simulink model "trajgen2_ste2_realtraj"  (R2016a)
settings: Solver=FixedStepDiscrete  StartTime=0.0  StopTime=10  RelTol=1e-3
undefined symbols (not defined in the file or in its folder): min_dist, robot_trajectory_data, robot_trajectory_s, start_time, THumanSingleTask
settings Model: Creator=ihout_000  LastModifiedBy=utente
settings DataIOCC: SaveFormat=Array
settings OptimizationCC: ExpressionDepthLimit=2147483647  SimCompilerOptimization=on
settings DebuggingCC: UnderspecifiedInitializationDetection=Classic  MergeDetectMultiDrivingBlocksExec=none  SolverPrmCheckMsg=warning  InheritedTsInSrcMsg=none  StateNameClashWarn=warning
settings HardwareCC: ProdBitPerPointer=32  ProdLargestAtomicFloat=None  ProdIntDivRoundTo=Undefined  ProdEndianess=Unspecified  ProdWordSize=32  ProdHWDeviceType=32-bit Generic
settings ModelReferenceCC: PropagateSignalLabelsOutOfModel=off
settings SFSimCC: SimUserIncludeDirs=ReflexxesTypeII\include\
settings SFSimCC: SimUserSources=|
  | ReflexxesTypeII\src\TypeIIRML\ReflexxesAPI.cpp
  | ReflexxesTypeII\src\TypeIIRML\TypeIIRMLCalculatePositionalExtrems.cpp
  | ReflexxesTypeII\src\TypeIIRML\TypeIIRMLDecisions.cpp
  | ReflexxesTypeII\src\TypeIIRML\TypeIIRMLDecisionTree1A.cpp
  | ReflexxesTypeII\src\TypeIIRML\TypeIIRMLDecisionTree1B.cpp
  | ReflexxesTypeII\src\TypeIIRML\TypeIIRMLDecisionTree1C.cpp
  | ReflexxesTypeII\src\TypeIIRML\TypeIIRMLDecisionTree2.cpp
  | ReflexxesTypeII\src\TypeIIRML\TypeIIRMLFallBackStrategy.cpp
  | ReflexxesTypeII\src\TypeIIRML\TypeIIRMLIsPhaseSynchronizationPossible.cpp
  | ReflexxesTypeII\src\TypeIIRML\TypeIIRMLPolynomial.cpp
  | ReflexxesTypeII\src\TypeIIRML\TypeIIRMLPosition.cpp
  | ReflexxesTypeII\src\TypeIIRML\TypeIIRMLQuicksort.cpp
  | ReflexxesTypeII\src\TypeIIRML\TypeIIRMLSetupModifiedSelectionVector.cpp
  | ReflexxesTypeII\src\TypeIIRML\TypeIIRMLStep1.cpp
  | ReflexxesTypeII\src\TypeIIRML\TypeIIRMLStep1IntermediateProfiles.cpp
  | ReflexxesTypeII\src\TypeIIRML\TypeIIRMLStep1Profiles.cpp
  | ReflexxesTypeII\src\TypeIIRML\TypeIIRMLStep2.cpp
  | ReflexxesTypeII\src\TypeIIRML\TypeIIRMLStep2IntermediateProfiles.cpp
  | ReflexxesTypeII\src\TypeIIRML\TypeIIRMLStep2PhaseSynchronization.cpp
  | ReflexxesTypeII\src\TypeIIRML\TypeIIRMLStep2Profiles.cpp
  | ReflexxesTypeII\src\TypeIIRML\TypeIIRMLStep2WithoutSynchronization.cpp
  | ReflexxesTypeII\src\TypeIIRML\TypeIIRMLStep3.cpp
  | ReflexxesTypeII\src\TypeIIRML\TypeIIRMLVelocity.cpp
  | ReflexxesTypeII\src\TypeIIRML\TypeIIRMLVelocityCalculatePositionalExtrems.cpp
  | ReflexxesTypeII\src\TypeIIRML\TypeIIRMLVelocityFallBackStrategy.cpp
  | ReflexxesTypeII\src\TypeIIRML\TypeIIRMLVelocityIsPhaseSynchronizationPossible.cpp
  | ReflexxesTypeII\src\TypeIIRML\TypeIIRMLVelocityMethods.cpp
  | ReflexxesTypeII\src\TypeIIRML\TypeIIRMLVelocitySetupPhaseSyncSelectionVector.cpp
settings RTWCC: GenerateMakefile=off  CustomInclude=ReflexxesTypeII\include\  TargetLang=C++  RTWCompilerOptimization=on
settings RTWCC: CustomSource=|
  | ReflexxesTypeII\src\TypeIIRML\ReflexxesAPI.cpp
  | ReflexxesTypeII\src\TypeIIRML\TypeIIRMLCalculatePositionalExtrems.cpp
  | ReflexxesTypeII\src\TypeIIRML\TypeIIRMLDecisions.cpp
  | ReflexxesTypeII\src\TypeIIRML\TypeIIRMLDecisionTree1A.cpp
  | ReflexxesTypeII\src\TypeIIRML\TypeIIRMLDecisionTree1B.cpp
  | ReflexxesTypeII\src\TypeIIRML\TypeIIRMLDecisionTree1C.cpp
  | ReflexxesTypeII\src\TypeIIRML\TypeIIRMLDecisionTree2.cpp
  | ReflexxesTypeII\src\TypeIIRML\TypeIIRMLFallBackStrategy.cpp
  | ReflexxesTypeII\src\TypeIIRML\TypeIIRMLIsPhaseSynchronizationPossible.cpp
  | ReflexxesTypeII\src\TypeIIRML\TypeIIRMLPolynomial.cpp
  | ReflexxesTypeII\src\TypeIIRML\TypeIIRMLPosition.cpp
  | ReflexxesTypeII\src\TypeIIRML\TypeIIRMLQuicksort.cpp
  | ReflexxesTypeII\src\TypeIIRML\TypeIIRMLSetupModifiedSelectionVector.cpp
  | ReflexxesTypeII\src\TypeIIRML\TypeIIRMLStep1.cpp
  | ReflexxesTypeII\src\TypeIIRML\TypeIIRMLStep1IntermediateProfiles.cpp
  | ReflexxesTypeII\src\TypeIIRML\TypeIIRMLStep1Profiles.cpp
  | ReflexxesTypeII\src\TypeIIRML\TypeIIRMLStep2.cpp
  | ReflexxesTypeII\src\TypeIIRML\TypeIIRMLStep2IntermediateProfiles.cpp
  | ReflexxesTypeII\src\TypeIIRML\TypeIIRMLStep2PhaseSynchronization.cpp
  | ReflexxesTypeII\src\TypeIIRML\TypeIIRMLStep2Profiles.cpp
  | ReflexxesTypeII\src\TypeIIRML\TypeIIRMLStep2WithoutSynchronization.cpp
  | ReflexxesTypeII\src\TypeIIRML\TypeIIRMLStep3.cpp
  | ReflexxesTypeII\src\TypeIIRML\TypeIIRMLVelocity.cpp
  | ReflexxesTypeII\src\TypeIIRML\TypeIIRMLVelocityCalculatePositionalExtrems.cpp
  | ReflexxesTypeII\src\TypeIIRML\TypeIIRMLVelocityFallBackStrategy.cpp
  | ReflexxesTypeII\src\TypeIIRML\TypeIIRMLVelocityIsPhaseSynchronizationPossible.cpp
  | ReflexxesTypeII\src\TypeIIRML\TypeIIRMLVelocityMethods.cpp
  | ReflexxesTypeII\src\TypeIIRML\TypeIIRMLVelocitySetupPhaseSyncSelectionVector.cpp
settings GRTTargetCC: TargetLangStandard=C++03 (ISO)
settings ConfigComp: CovModelRefEnable=Off

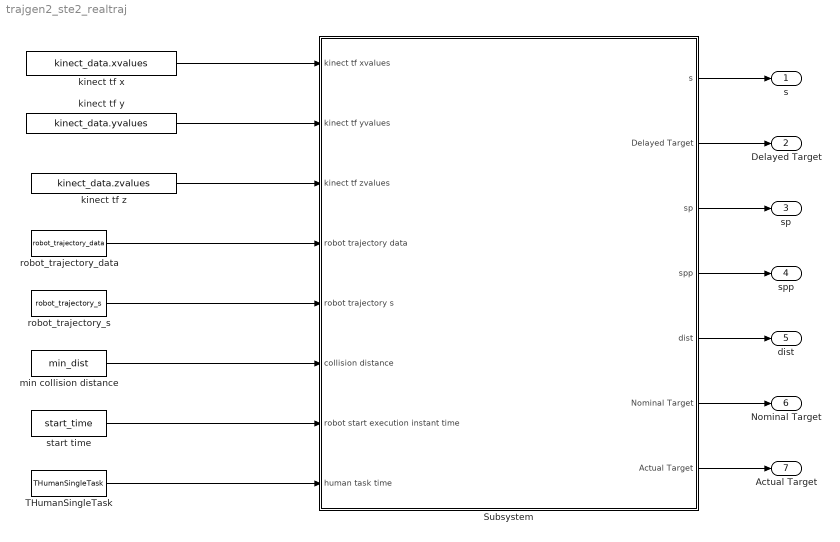
== system trajgen2_ste2_realtraj ==
  Subsystem : Subsystem
  THumanSingleTask : Constant  Value=THumanSingleTask
  kinect tf x : FromWorkspace  VariableName=kinect_data.xvalues  OutDataTypeStr=double
  kinect tf y : FromWorkspace  VariableName=kinect_data.yvalues  SampleTime=0
  kinect tf z : FromWorkspace  VariableName=kinect_data.zvalues  SampleTime=0
  min collision distance : Constant  Value=min_dist
  robot_trajectory_data : Constant  Value=robot_trajectory_data
  robot_trajectory_s : Constant  Value=robot_trajectory_s
  start time : Constant  Value=start_time
  s : Outport
  "Delayed Target " : Outport  Port=2
  sp : Outport  Port=3
  spp : Outport  Port=4
  dist : Outport  Port=5
  Nominal Target : Outport  Port=6
  Actual Target : Outport  Port=7
  wires:
  Subsystem/1(s) -> s/1
  kinect tf x/1 -> Subsystem/1("kinect tf xvalues ")
  kinect tf z/1 -> Subsystem/3(kinect tf zvalues)
  kinect tf y/1 -> Subsystem/2(kinect tf yvalues)
  Subsystem/2("Delayed Target ") -> "Delayed Target "/1
  robot_trajectory_data/1 -> Subsystem/4(robot trajectory data)
  robot_trajectory_s/1 -> Subsystem/5(robot trajectory s)
  Subsystem/5(dist) -> dist/1
  Subsystem/3(sp) -> sp/1
  Subsystem/4(spp) -> spp/1
  min collision distance/1 -> Subsystem/6(collision distance)
  Subsystem/6(Nominal Target) -> Nominal Target/1
  Subsystem/7(Actual Target) -> Actual Target/1
  start time/1 -> Subsystem/7(robot start execution instant time)
  THumanSingleTask/1 -> Subsystem/8("human task time ")

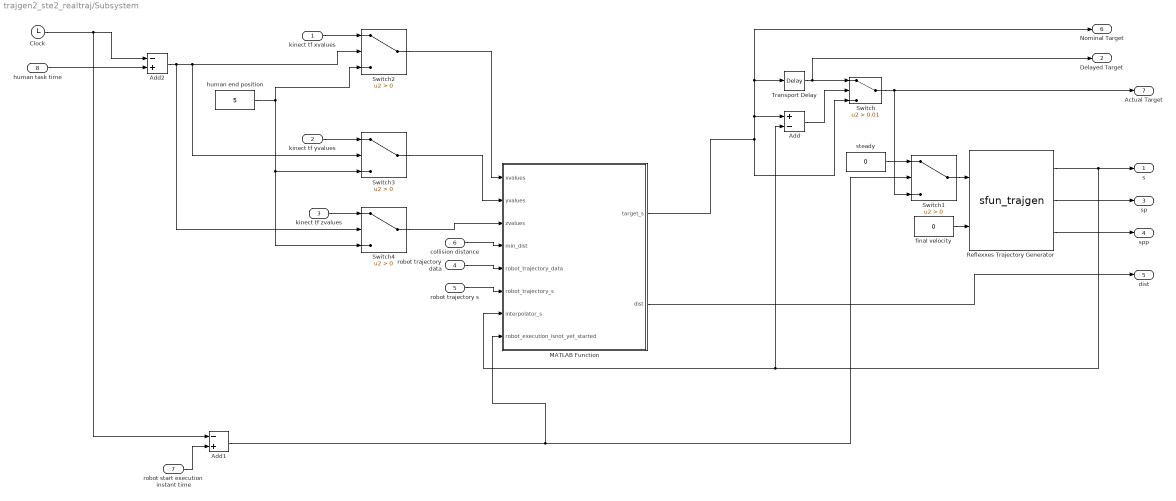
== system trajgen2_ste2_realtraj/Subsystem ==
  "kinect tf xvalues " : Inport
  kinect tf yvalues : Inport  Port=2
  kinect tf zvalues : Inport  Port=3
  robot trajectory data : Inport  Port=4
  robot trajectory s : Inport  Port=5
  collision distance : Inport  Port=6
  robot start execution instant time : Inport  Port=7
  "human task time " : Inport  Port=8
  Add : Sum  Inputs=+-
  Add1 : Sum  Inputs=-+
  Add2 : Sum  Inputs=-+
  Clock : Clock
  MATLAB Function : MATLAB Function  TreatAsAtomicUnit=on
  Reflexxes Trajectory Generator : S-Function  FunctionName=sfun_trajgen  Parameters=ts,ndofs,pinit,vmax,amax,jmax,sync  SFunctionDeploymentMode=off  EnableBusSupport=off  mask{ts=0.005, ndofs=1, pinit=0, vmax=0.250, amax=0.115, jmax=10000000000, sync=PHASE_SYNCHRONIZATION_IF_POSSIBLE}
      mask prompts: ts "Sample Time:"; ndofs "Number of DoF's:"; pinit "Initial Position Vector:"; vmax "Maximum Velocity Vector:"; amax "Maximum Acceleration Vector:"; jmax "Maximum Jerk Vector:"; sync "Synchronization Behavior:"
      mask TypeOptions sync: NO_SYNCHRONIZATION | PHASE_SYNCHRONIZATION_IF_POSSIBLE | ONLY_TIME_SYNCHRONIZATION | ONLY_PHASE_SYNCHRONIZATION
      mask Display:
      | port_label('input', 1, 'target_pos')
      | port_label('input', 2, 'target_vel')
      | port_label('output', 1, 'pos')
      | port_label('output', 2, 'vel')
      | port_label('output', 3, 'acc')
  Switch : Switch  Criteria=u2 > Threshold  Threshold=0.01
  Switch{1..4} (4 alike) : Switch  Criteria=u2 > Threshold
  Transport Delay : TransportDelay  DelayTime=0.5
  final velocity : Constant  Value=0
  human end position : Constant  Value=5
  steady : Constant  Value=0
  s : Outport
  "Delayed Target " : Outport  Port=2
  sp : Outport  Port=3
  spp : Outport  Port=4
  dist : Outport  Port=5
  Nominal Target : Outport  Port=6
  Actual Target : Outport  Port=7
  wires:
  Reflexxes Trajectory Generator/1 -> Add/2, MATLAB Function/7(interpolator_s), s/1
  final velocity/1 -> Reflexxes Trajectory Generator/2
  kinect tf yvalues/1 -> Switch3/1
  kinect tf zvalues/1 -> Switch4/1
  MATLAB Function/1(target_s) -> Nominal Target/1, Transport Delay/1, Add/1, Switch/3
  robot trajectory data/1 -> MATLAB Function/5(robot_trajectory_data)
  robot trajectory s/1 -> MATLAB Function/6(robot_trajectory_s)
  MATLAB Function/2(dist) -> dist/1
  Reflexxes Trajectory Generator/2 -> sp/1
  Reflexxes Trajectory Generator/3 -> spp/1
  collision distance/1 -> MATLAB Function/4(min_dist)
  Switch/1 -> Switch1/3, Actual Target/1
  Transport Delay/1 -> "Delayed Target "/1, Switch/1
  Add/1 -> Switch/2
  Switch1/1 -> Reflexxes Trajectory Generator/1
  robot start execution instant time/1 -> Add1/2
  Add1/1 -> Switch1/2, MATLAB Function/8(robot_execution_isnot_yet_started)
  steady/1 -> Switch1/1
  "kinect tf xvalues "/1 -> Switch2/1
  "human task time "/1 -> Add2/2
  Clock/1 -> Add1/1, Add2/1
  Add2/1 -> Switch4/2, Switch3/2, Switch2/2
  human end position/1 -> Switch2/3, Switch3/3, Switch4/3
  Switch2/1 -> MATLAB Function/1(xvalues)
  Switch3/1 -> MATLAB Function/2(yvalues)
  Switch4/1 -> MATLAB Function/3(zvalues)

== matlab function trajgen2_ste2_realtraj/Subsystem/MATLAB Function ==
  data: xvalues input; yvalues input; zvalues input; min_dist input; robot_trajectory_data input; robot_trajectory_s input; interpolator_s input; robot_execution_isnot_yet_started input; target_s output; dist output
function [ target_s, dist] = fcn( xvalues, yvalues, zvalues, min_dist, robot_trajectory_data, robot_trajectory_s, interpolator_s, robot_execution_isnot_yet_started )

coder.extrinsic('diff');
coder.extrinsic('cumsum');

persistent speex speey speez spwx spwy spwz spex spey spez dex dey dez de deex deey deez dee dwx dwy dwz dw dlx dly dlz dl

if isempty( speex )
    % spline end-effector
    speex = spline( robot_trajectory_s, robot_trajectory_data(:,1) );
    speey = spline( robot_trajectory_s, robot_trajectory_data(:,2) );
    speez = spline( robot_trajectory_s, robot_trajectory_data(:,3) );

    % spline wrist
    spwx  = spline( robot_trajectory_s, robot_trajectory_data(:,4) );
    spwy  = spline( robot_trajectory_s, robot_trajectory_data(:,5) );
    spwz  = spline( robot_trajectory_s, robot_trajectory_data(:,6) );

    % spline elbow
    spex  = spline( robot_trajectory_s, robot_trajectory_data(:,7) );
    spey  = spline( robot_trajectory_s, robot_trajectory_data(:,8) );
    spez  = spline( robot_trajectory_s, robot_trajectory_data(:,9) );
    
    dex  = 0; dey  = 0; dez  = 0; de  = 0;
    dwx  = 0; dwy  = 0; dwz  = 0; dw  = 0;
    deex = 0; deey = 0; deez = 0; dee = 0;
    dlx  = 0; dly  = 0; dlz  = 0; dl  = 0;

end

%%% pos end-effector
ree = [ ppval( interpolator_s * robot_trajectory_s(end), speex )' ... 
      ; ppval( interpolator_s * robot_trajectory_s(end), speey )' ...
      ; ppval( interpolator_s * robot_trajectory_s(end), speez )' ];

%%% pos wrist
rw  = [ ppval( interpolator_s * robot_trajectory_s(end), spwx )' ... 
      ; ppval( interpolator_s * robot_trajectory_s(end), spwy )' ...
      ; ppval( interpolator_s * robot_trajectory_s(end), spwz )' ];

%%% pos elbow
re  = [ ppval( interpolator_s * robot_trajectory_s(end), spex )' ... 
      ; ppval( interpolator_s * robot_trajectory_s(end), spey )' ...
      ; ppval( interpolator_s * robot_trajectory_s(end), spez )' ];

%%% each value is corresponding to the xyz of a different tf
dist = 0;
if (robot_execution_isnot_yet_started >= 0)
    target_s = 0;
elseif interpolator_s == 1
    target_s = interpolator_s;
else 
    for i=1:length(xvalues) %%% cycle over tf

        % distance human - ee
        deex = xvalues(i) - ree(1); deey = yvalues(i) - ree(2); deez = zvalues(i) - ree(3);
        dee  = sqrt( deex^2 + deey^2 + deez^2 ); 
        
        % distance human - wrist
        dwx  = xvalues(i) - rw(1);  dwy  = yvalues(i) - rw(2);  dwz  = zvalues(i) - rw(3);
        dw   = sqrt( dwx^2  + dwy^2  + dwz^2  );
        
        % distance human - elbow
        dex  = xvalues(i) - re(1);  dey  = yvalues(i) - re(2);  dez  = zvalues(i) - re(3);
        de   = sqrt( dex^2  + dey^2  + dez^2  );
        
        % distance human - line from elbow to wrsit
        dwex = rw(1)-re(1);  dwey  = (rw(2) - re(2) );  dwez  = (rw(3) - re(3) );

        dlx  = (  dey*dwez - dez*dwey ) / sqrt( dwex^2 + dwey^2 + dwez^2 );
        dly  = (  dez*dwex - dex*dwez ) / sqrt( dwex^2 + dwey^2 + dwez^2 );
        dlz  = (  dex*dwey - dey*dwex ) / sqrt( dwex^2 + dwey^2 + dwez^2 );
        
        dl   = sqrt( dlx^2 + dly^2 + dlz^2 );
        
        dist = min( [dee, dw, de, dl ] ) ;
        
        if dist > min_dist
            target_s = 1;
        else
            target_s = interpolator_s;
            break;
        end
    end
end

 %target_s = 1;
